simulink model "Kalman_fil"  (R2018a)
settings: Solver=VariableStepAuto  StartTime=0.0  StopTime=10.0  RelTol=1e-3
values from neighbouring files (symbols this model uses):
  A = [[1 dt];[0 (1+(k/m)*dt) ]]    [Model.m]    (also in Parameter.m; Three_phase_Kalman_Parameter.m = [1 0; 0 a22])
  B = [[1 0];[0 -g*dt]]    [Model.m]    (also in Parameter.m)
  C = eye(2)    [Parameter.m]    (also in Three_phase_Kalman_Parameter.m = [1 1])
  D = 0    [Parameter.m]
  dt = 0.01    [Model.m]    (also in Parameter.m)
  g = 9.8    [Model.m]    (also in Parameter.m)
  k = -1.0    (= -1)    [Model.m]    (also in Parameter.m)
  m = 1.0    (= 1)    [Model.m]    (also in Parameter.m)
  MNV = MNstd*MNstd    (= 0.16)    [Parameter.m]
  PNV = PNstd*PNstd    (= 0.0004)    [Parameter.m]
  R = eye(2)*MNV    [Parameter.m]    (also in Three_phase_Kalman_Parameter.m = 25)
  Ts = dt    (= 0.01)    [Parameter.m]    (also in Three_phase_Kalman_Parameter.m = 0.0001)
undefined symbols (not defined in the file or in its folder): Discrete, Time
libraries: ctrlSharedLib x1
settings Model: Creator=User  LastModifiedBy=User

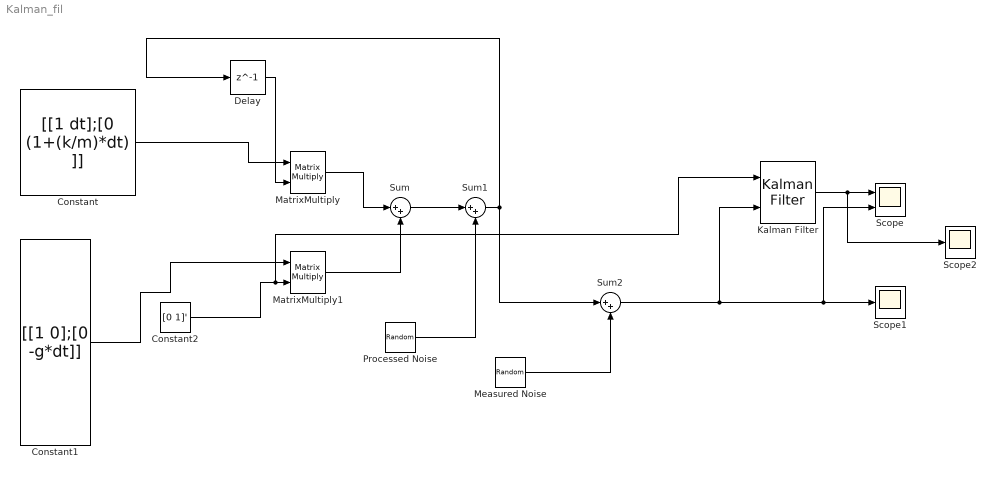
== system Kalman_fil ==
  Constant : Constant  Value=[[1 dt];[0 (1+(k/m)*dt) ]]
  Constant1 : Constant  Value=[[1 0];[0 -g*dt]]
  Constant2 : Constant  Value=[0 1]'
  Delay : Delay  DelayLength=1
  Kalman Filter : ctrlSharedLib/Kalman Filter  TimeDomain=Discrete-Time  UseCurrentEstimator=on  ModelSource=Individual A, B, C, D matrices  ModelSourceVariable=ss(0.95,1,1,0,1)  A=A  B=B  C=C  D=D  NumberOfStates=1  NumberOfInputs=1  NumberOfOutputs=1  InitialEstimateSource=Dialog  X0=[0;0]  P0=10  UseK=off  UseGH=off  NumberOfProcessNoiseInputs=1  G=1  TimeInvariantG=on  H=0  TimeInvariantH=on  Q=Q  TimeInvariantQ=on  R=R  TimeInvariantR=on  N=0  TimeInvariantN=on  AddInputPort=on  AddEnablePort=off  OutputEstimatedY=off  OutputP=off  Ts=Ts
      settings: SourceProductBaseCode=CT
  MatrixMultiply : Product  Multiplication=Matrix(*)
  MatrixMultiply1 : Product  Multiplication=Matrix(*)
  "Measured Noise " : RandomNumber  Variance=MNV  Seed=[23341]  SampleTime=Ts
  Processed Noise : RandomNumber  Variance=PNV  Seed=[23341]  SampleTime=Ts
  Scope : Scope  NumInputPorts=2
  Scope1 : Scope
  Scope2 : Scope
  Sum : Sum  Inputs=|++
  Sum1 : Sum  Inputs=|++
  Sum2 : Sum  Inputs=|++
  wires:
  Constant/1 -> MatrixMultiply/1
  Delay/1 -> MatrixMultiply/2
  Constant1/1 -> MatrixMultiply1/1
  Constant2/1 -> Kalman Filter/1, MatrixMultiply1/2
  MatrixMultiply/1 -> Sum/1
  MatrixMultiply1/1 -> Sum/2
  Processed Noise/1 -> Sum1/2
  Sum/1 -> Sum1/1
  Sum1/1 -> Sum2/1, Delay/1
  "Measured Noise "/1 -> Sum2/2
  Sum2/1 -> Scope/2, Scope1/1, Kalman Filter/2
  Kalman Filter/1 -> Scope2/1, Scope/1
